simulink library "interface_to_SPS_from_Simulink_lib_2011"  (Simulink 7.8)
settings: Solver=ode45  StartTime=0.0  StopTime=10.0  RelTol=1e-3
libraries: powerlib x6
settings Model: Creator=CH24070  LastModifiedBy=CH24070

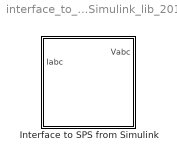
== system interface_to_SPS_from_Simulink_lib_2011 ==
  Interface to SPS from Simulink : Subsystem

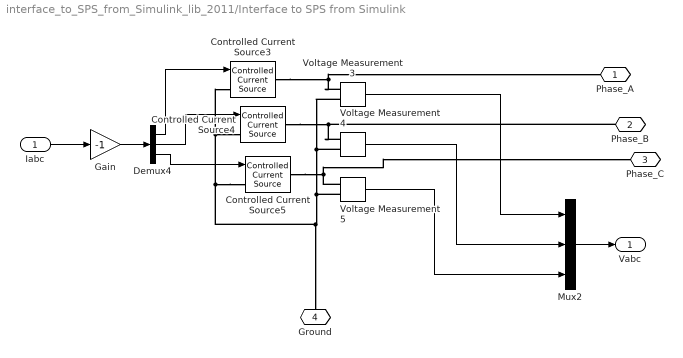
== system interface_to_SPS_from_Simulink_lib_2011/Interface to SPS from Simulink ==
  Iabc : Inport
  Controlled Current Source3 : powerlib/Electrical Sources/Controlled Current Source  Initialize=on  Source_Type=AC  Amplitude=0  Phase=0  Frequency=0  Measurements=None
  Controlled Current Source4 : powerlib/Electrical Sources/Controlled Current Source  Initialize=on  Source_Type=AC  Amplitude=0  Phase=0  Frequency=0  Measurements=None
  Controlled Current Source5 : powerlib/Electrical Sources/Controlled Current Source  Initialize=on  Source_Type=AC  Amplitude=0  Phase=0  Frequency=0  Measurements=None
  Demux4 : Demux  Outputs=3
  Gain : Gain  Gain=-1
  Mux2 : Mux  Inputs=3
  Voltage Measurement3 : powerlib/Measurements/Voltage Measurement  PhasorSimulation=off  OutputType=Complex  PSBequivalent=0
  Voltage Measurement4 : powerlib/Measurements/Voltage Measurement  PhasorSimulation=off  OutputType=Complex  PSBequivalent=0
  Voltage Measurement5 : powerlib/Measurements/Voltage Measurement  PhasorSimulation=off  OutputType=Complex  PSBequivalent=0
  Phase_A : PMIOPort  Port=1  Side=Right
  Phase_B : PMIOPort  Port=2  Side=Right
  Phase_C : PMIOPort  Port=3  Side=Right
  Ground : PMIOPort  Port=4  Side=Left
  Vabc : Outport
  wires:
  Voltage Measurement5/1 -> Mux2/3
  Voltage Measurement4/1 -> Mux2/2
  Demux4/1 -> Controlled Current Source3/1
  Demux4/2 -> Controlled Current Source4/1
  Demux4/3 -> Controlled Current Source5/1
  Iabc/1 -> Gain/1
  Mux2/1 -> Vabc/1
  Voltage Measurement3/1 -> Mux2/1
  Gain/1 -> Demux4/1
  connections:
  Voltage Measurement5/LConn1 -- Controlled Current Source5/RConn1 -- Phase_C/RConn1
  Voltage Measurement3/LConn1 -- Controlled Current Source3/RConn1 -- Phase_A/RConn1
  Controlled Current Source5/LConn1 -- Controlled Current Source3/LConn1 -- Controlled Current Source4/LConn1 -- Voltage Measurement4/LConn2 -- Voltage Measurement3/LConn2 -- Voltage Measurement5/LConn2 -- Ground/RConn1
  Voltage Measurement4/LConn1 -- Controlled Current Source4/RConn1 -- Phase_B/RConn1
